simulink model "CubeSat_Archiv"  (R2019a)
settings: Solver=VariableStepAuto  StartTime=0.0  StopTime=10.0  RelTol=1e-3
undefined symbols (not defined in the file): D_distri, G_g, G_s, G_t, Gs, I_rw, I_vscmg, I_w, J_w, Kc, Ki, Kp, Kv, Kw_d, Kw_i, Kw_p, m, OMEGA_0, quat_0, smiData, tau_sat_mt, w_rw_ref, X, Y, Z
libraries: sm_lib x57, nesl_utility x28, aerolibutil x18, sharedtransform x5, ADCS_lib x4, simulink x2, sharedutil x2
(part 4 of 4)

== system CubeSat_Archiv/Simscape Plant/Simscape Plant1/CubeSat Structure ==
  BODY_FIXED_CoMXform : sm_lib/Frames and Transforms/Rigid Transform  TranslationMethod=Cartesian  TranslationStandardOffset=0  TranslationLengthUnit=mm  TranslationStandardAxis=+Z  TranslationCartesianOffset=smiData.RigidTransform(10).translation  TranslationROffset=0  TranslationROffsetUnits=m  TranslationZOffset=0  TranslationZOffsetUnits=m  TranslationThetaOffset=0  TranslationThetaOffsetUnits=deg  RotationMethod=ArbitraryAxis  RotationAngleUnits=rad  RotationStandardAxis=+Z  RotationAngle=smiData.RigidTransform(10).angle  RotationArbitraryAxis=smiData.RigidTransform(10).axis  FollAlignAxisA=+X  BaseAlignAxisA=+Y  FollAlignAxisB=+Y  BaseAlignAxisB=+Z  RotationSequenceAxes=FollowerAxes  RotationSequence=XYX  RotationSequenceAngles=[0 0 0]  RotationSequenceAnglesUnits=deg  RotationMatrix=[1 0 0; 0 1 0; 0 0 1]
  ReferenceFrame : sm_lib/Frames and Transforms/Reference Frame
  Solid : sm_lib/Body Elements/Solid  InertiaType=Custom  Mass=smiData.Solid(1).mass  MassUnits=kg  CenterOfMass=smiData.Solid(1).CoM  CenterOfMassUnits=mm  MomentsOfInertia=smiData.Solid(1).MoI  MomentsOfInertiaUnits=kg*mm^2  ProductsOfInertia=smiData.Solid(1).PoI  ProductsOfInertiaUnits=kg*mm^2  BasedOnType=Density  Density=1000  DensityUnits=kg/m^3  DoExposeReferenceFrame=on  SerializedFrames=<Frames><Frame><Id>Frame1</Id><Value><Name>F1</Name><Origin><Source>CenterOfMassFrame</Source><FeatureName></FeatureName></Origin><PrimaryAxis><DefinedDirection>+Z</DefinedDirection><Source>ReferenceFrame</Source><SourceDirection>+Z</SourceDirection><FeatureName></FeatureName></PrimaryAxis><SecondaryAxis><DefinedDirection>+X</DefinedDirection><Source>ReferenceFrame</Source><SourceDirection>+X</SourceDirection><FeatureName></FeatureName></SecondaryAxis></Value></Frame></Frames>  GraphicType=FromGeometry  MarkerShape=Sphere  MarkerSize=10  GraphicVisPropType=SimpleVisualProperties  GraphicDiffuseColor=[0.6 0.6 0.6]  GraphicSpecularColor=[0.5 0.5 0.5 1.0]  GraphicAmbientColor=[0.15 0.15 0.15 1.0]  GraphicEmissiveColor=[0.0 0.0 0.0 1.0]  GraphicShininess=100  GraphicOpacity=smiData.Solid(1).opacity  GeometryShape=FromFile  RectangleSize=[1 1]  RectangleSizeUnits=m  BrickDimensions=[1 1 1]  BrickDimensionUnits=m  CylinderRadius=1  CylinderRadiusUnits=m  CylinderLength=1  CylinderLengthUnits=m  SphereRadius=1  SphereRadiusUnits=m  EllipsoidRadii=[1 1 1]  EllipsoidRadiiUnits=m  ExtrusionCrossSection=[1 1; -1 1; -1 -1; 1 -1]  ExtrusionCrossSectionUnits=m  ExtrusionLength=1  ExtrusionLengthUnits=m  PolygonNumSides=3  PolygonOuterRadius=1  PolygonOuterRadiusUnits=m  ExtGeomFileType=STEP  ExtGeomFileName=body_part_acis_Default_sldprt.STEP  ExtGeomFileUnits=m  RevolutionCrossSection=[1 1; 1 -1; 2 -1; 2 1]  RevolutionCrossSectionUnits=m  RevolutionExtent=Full  RevolutionAngle=180  RevolutionAngleUnits=deg
  Transform : sm_lib/Frames and Transforms/Rigid Transform  TranslationMethod=Cartesian  TranslationStandardOffset=0  TranslationLengthUnit=mm  TranslationStandardAxis=+Z  TranslationCartesianOffset=smiData.RigidTransform(1).translation  TranslationROffset=0  TranslationROffsetUnits=m  TranslationZOffset=0  TranslationZOffsetUnits=m  TranslationThetaOffset=0  TranslationThetaOffsetUnits=deg  RotationMethod=ArbitraryAxis  RotationAngleUnits=rad  RotationStandardAxis=+Z  RotationAngle=smiData.RigidTransform(1).angle  RotationArbitraryAxis=smiData.RigidTransform(1).axis  FollAlignAxisA=+X  BaseAlignAxisA=+Y  FollAlignAxisB=+Y  BaseAlignAxisB=+Z  RotationSequenceAxes=FollowerAxes  RotationSequence=XYX  RotationSequenceAngles=[0 0 0]  RotationSequenceAnglesUnits=deg  RotationMatrix=[1 0 0; 0 1 0; 0 0 1]
  Transform1 : sm_lib/Frames and Transforms/Rigid Transform  TranslationMethod=Cartesian  TranslationStandardOffset=0  TranslationLengthUnit=mm  TranslationStandardAxis=+Z  TranslationCartesianOffset=smiData.RigidTransform(3).translation  TranslationROffset=0  TranslationROffsetUnits=m  TranslationZOffset=0  TranslationZOffsetUnits=m  TranslationThetaOffset=0  TranslationThetaOffsetUnits=deg  RotationMethod=ArbitraryAxis  RotationAngleUnits=rad  RotationStandardAxis=+Z  RotationAngle=smiData.RigidTransform(3).angle  RotationArbitraryAxis=smiData.RigidTransform(3).axis  FollAlignAxisA=+X  BaseAlignAxisA=+Y  FollAlignAxisB=+Y  BaseAlignAxisB=+Z  RotationSequenceAxes=FollowerAxes  RotationSequence=XYX  RotationSequenceAngles=[0 0 0]  RotationSequenceAnglesUnits=deg  RotationMatrix=[1 0 0; 0 1 0; 0 0 1]
  Transform2 : sm_lib/Frames and Transforms/Rigid Transform  TranslationMethod=Cartesian  TranslationStandardOffset=0  TranslationLengthUnit=mm  TranslationStandardAxis=+Z  TranslationCartesianOffset=smiData.RigidTransform(5).translation  TranslationROffset=0  TranslationROffsetUnits=m  TranslationZOffset=0  TranslationZOffsetUnits=m  TranslationThetaOffset=0  TranslationThetaOffsetUnits=deg  RotationMethod=ArbitraryAxis  RotationAngleUnits=rad  RotationStandardAxis=+Z  RotationAngle=smiData.RigidTransform(5).angle  RotationArbitraryAxis=smiData.RigidTransform(5).axis  FollAlignAxisA=+X  BaseAlignAxisA=+Y  FollAlignAxisB=+Y  BaseAlignAxisB=+Z  RotationSequenceAxes=FollowerAxes  RotationSequence=XYX  RotationSequenceAngles=[0 0 0]  RotationSequenceAnglesUnits=deg  RotationMatrix=[1 0 0; 0 1 0; 0 0 1]
  Transform3 : sm_lib/Frames and Transforms/Rigid Transform  TranslationMethod=Cartesian  TranslationStandardOffset=0  TranslationLengthUnit=mm  TranslationStandardAxis=+Z  TranslationCartesianOffset=smiData.RigidTransform(7).translation  TranslationROffset=0  TranslationROffsetUnits=m  TranslationZOffset=0  TranslationZOffsetUnits=m  TranslationThetaOffset=0  TranslationThetaOffsetUnits=deg  RotationMethod=ArbitraryAxis  RotationAngleUnits=rad  RotationStandardAxis=+Z  RotationAngle=smiData.RigidTransform(7).angle  RotationArbitraryAxis=smiData.RigidTransform(7).axis  FollAlignAxisA=+X  BaseAlignAxisA=+Y  FollAlignAxisB=+Y  BaseAlignAxisB=+Z  RotationSequenceAxes=FollowerAxes  RotationSequence=XYX  RotationSequenceAngles=[0 0 0]  RotationSequenceAnglesUnits=deg  RotationMatrix=[1 0 0; 0 1 0; 0 0 1]
  CoM : PMIOPort  Side=Left
  F3 : PMIOPort  Port=2  Side=Right
  F2 : PMIOPort  Port=3  Side=Right
  F1 : PMIOPort  Port=4  Side=Right
  F : PMIOPort  Port=5  Side=Right
  connections:
  BODY_FIXED_CoMXform/LConn1 -- CoM/RConn1
  Transform3/RConn1 -- F3/RConn1
  Transform2/RConn1 -- F2/RConn1
  Transform1/RConn1 -- F1/RConn1
  Transform/RConn1 -- F/RConn1
  Transform2/LConn1 -- BODY_FIXED_CoMXform/RConn1 -- Transform3/LConn1 -- ReferenceFrame/RConn1 -- Solid/RConn1 -- Transform1/LConn1 -- Transform/LConn1

== system CubeSat_Archiv/Simscape Plant/Simscape Plant1/RW 1 Disk ==
  ReferenceFrame : sm_lib/Frames and Transforms/Reference Frame
  Solid : sm_lib/Body Elements/Solid  InertiaType=Custom  Mass=smiData.Solid(2).mass  MassUnits=kg  CenterOfMass=smiData.Solid(2).CoM  CenterOfMassUnits=mm  MomentsOfInertia=smiData.Solid(2).MoI  MomentsOfInertiaUnits=kg*mm^2  ProductsOfInertia=smiData.Solid(2).PoI  ProductsOfInertiaUnits=kg*mm^2  BasedOnType=Density  Density=1000  DensityUnits=kg/m^3  DoExposeReferenceFrame=on  SerializedFrames=<Frames/>  GraphicType=FromGeometry  MarkerShape=Sphere  MarkerSize=10  GraphicVisPropType=SimpleVisualProperties  GraphicDiffuseColor=smiData.Solid(2).color  GraphicSpecularColor=[0.5 0.5 0.5 1.0]  GraphicAmbientColor=[0.15 0.15 0.15 1.0]  GraphicEmissiveColor=[0.0 0.0 0.0 1.0]  GraphicShininess=75  GraphicOpacity=smiData.Solid(2).opacity  GeometryShape=FromFile  RectangleSize=[1 1]  RectangleSizeUnits=m  BrickDimensions=[1 1 1]  BrickDimensionUnits=m  CylinderRadius=1  CylinderRadiusUnits=m  CylinderLength=1  CylinderLengthUnits=m  SphereRadius=1  SphereRadiusUnits=m  EllipsoidRadii=[1 1 1]  EllipsoidRadiiUnits=m  ExtrusionCrossSection=[1 1; -1 1; -1 -1; 1 -1]  ExtrusionCrossSectionUnits=m  ExtrusionLength=1  ExtrusionLengthUnits=m  PolygonNumSides=3  PolygonOuterRadius=1  PolygonOuterRadiusUnits=m  ExtGeomFileType=STEP  ExtGeomFileName=wheel_part_acis_Default_sldprt.STEP  ExtGeomFileUnits=m  RevolutionCrossSection=[1 1; 1 -1; 2 -1; 2 1]  RevolutionCrossSectionUnits=m  RevolutionExtent=Full  RevolutionAngle=180  RevolutionAngleUnits=deg
  Transform : sm_lib/Frames and Transforms/Rigid Transform  TranslationMethod=Cartesian  TranslationStandardOffset=0  TranslationLengthUnit=mm  TranslationStandardAxis=+Z  TranslationCartesianOffset=smiData.RigidTransform(4).translation  TranslationROffset=0  TranslationROffsetUnits=m  TranslationZOffset=0  TranslationZOffsetUnits=m  TranslationThetaOffset=0  TranslationThetaOffsetUnits=deg  RotationMethod=ArbitraryAxis  RotationAngleUnits=rad  RotationStandardAxis=+Z  RotationAngle=smiData.RigidTransform(4).angle  RotationArbitraryAxis=smiData.RigidTransform(4).axis  FollAlignAxisA=+X  BaseAlignAxisA=+Y  FollAlignAxisB=+Y  BaseAlignAxisB=+Z  RotationSequenceAxes=FollowerAxes  RotationSequence=XYX  RotationSequenceAngles=[0 0 0]  RotationSequenceAnglesUnits=deg  RotationMatrix=[1 0 0; 0 1 0; 0 0 1]
  F : PMIOPort  Side=Left
  connections:
  Transform/RConn1 -- F/RConn1
  Transform/LConn1 -- Solid/RConn1 -- ReferenceFrame/RConn1

== system CubeSat_Archiv/Simscape Plant/Simscape Plant1/RW 2 Disk ==
  ReferenceFrame : sm_lib/Frames and Transforms/Reference Frame
  Solid : sm_lib/Body Elements/Solid  InertiaType=Custom  Mass=smiData.Solid(2).mass  MassUnits=kg  CenterOfMass=smiData.Solid(2).CoM  CenterOfMassUnits=mm  MomentsOfInertia=smiData.Solid(2).MoI  MomentsOfInertiaUnits=kg*mm^2  ProductsOfInertia=smiData.Solid(2).PoI  ProductsOfInertiaUnits=kg*mm^2  BasedOnType=Density  Density=1000  DensityUnits=kg/m^3  DoExposeReferenceFrame=on  SerializedFrames=<Frames/>  GraphicType=FromGeometry  MarkerShape=Sphere  MarkerSize=10  GraphicVisPropType=SimpleVisualProperties  GraphicDiffuseColor=smiData.Solid(2).color  GraphicSpecularColor=[0.5 0.5 0.5 1.0]  GraphicAmbientColor=[0.15 0.15 0.15 1.0]  GraphicEmissiveColor=[0.0 0.0 0.0 1.0]  GraphicShininess=75  GraphicOpacity=smiData.Solid(2).opacity  GeometryShape=FromFile  RectangleSize=[1 1]  RectangleSizeUnits=m  BrickDimensions=[1 1 1]  BrickDimensionUnits=m  CylinderRadius=1  CylinderRadiusUnits=m  CylinderLength=1  CylinderLengthUnits=m  SphereRadius=1  SphereRadiusUnits=m  EllipsoidRadii=[1 1 1]  EllipsoidRadiiUnits=m  ExtrusionCrossSection=[1 1; -1 1; -1 -1; 1 -1]  ExtrusionCrossSectionUnits=m  ExtrusionLength=1  ExtrusionLengthUnits=m  PolygonNumSides=3  PolygonOuterRadius=1  PolygonOuterRadiusUnits=m  ExtGeomFileType=STEP  ExtGeomFileName=wheel_part_acis_Default_sldprt.STEP  ExtGeomFileUnits=m  RevolutionCrossSection=[1 1; 1 -1; 2 -1; 2 1]  RevolutionCrossSectionUnits=m  RevolutionExtent=Full  RevolutionAngle=180  RevolutionAngleUnits=deg
  Transform : sm_lib/Frames and Transforms/Rigid Transform  TranslationMethod=Cartesian  TranslationStandardOffset=0  TranslationLengthUnit=mm  TranslationStandardAxis=+Z  TranslationCartesianOffset=smiData.RigidTransform(6).translation  TranslationROffset=0  TranslationROffsetUnits=m  TranslationZOffset=0  TranslationZOffsetUnits=m  TranslationThetaOffset=0  TranslationThetaOffsetUnits=deg  RotationMethod=ArbitraryAxis  RotationAngleUnits=rad  RotationStandardAxis=+Z  RotationAngle=smiData.RigidTransform(6).angle  RotationArbitraryAxis=smiData.RigidTransform(6).axis  FollAlignAxisA=+X  BaseAlignAxisA=+Y  FollAlignAxisB=+Y  BaseAlignAxisB=+Z  RotationSequenceAxes=FollowerAxes  RotationSequence=XYX  RotationSequenceAngles=[0 0 0]  RotationSequenceAnglesUnits=deg  RotationMatrix=[1 0 0; 0 1 0; 0 0 1]
  F : PMIOPort  Side=Left
  connections:
  Transform/RConn1 -- F/RConn1
  Transform/LConn1 -- Solid/RConn1 -- ReferenceFrame/RConn1

== system CubeSat_Archiv/Simscape Plant/Simscape Plant1/RW 3 Disk ==
  ReferenceFrame : sm_lib/Frames and Transforms/Reference Frame
  Solid : sm_lib/Body Elements/Solid  InertiaType=Custom  Mass=smiData.Solid(2).mass  MassUnits=kg  CenterOfMass=smiData.Solid(2).CoM  CenterOfMassUnits=mm  MomentsOfInertia=smiData.Solid(2).MoI  MomentsOfInertiaUnits=kg*mm^2  ProductsOfInertia=smiData.Solid(2).PoI  ProductsOfInertiaUnits=kg*mm^2  BasedOnType=Density  Density=1000  DensityUnits=kg/m^3  DoExposeReferenceFrame=on  SerializedFrames=<Frames/>  GraphicType=FromGeometry  MarkerShape=Sphere  MarkerSize=10  GraphicVisPropType=SimpleVisualProperties  GraphicDiffuseColor=smiData.Solid(2).color  GraphicSpecularColor=[0.5 0.5 0.5 1.0]  GraphicAmbientColor=[0.15 0.15 0.15 1.0]  GraphicEmissiveColor=[0.0 0.0 0.0 1.0]  GraphicShininess=75  GraphicOpacity=smiData.Solid(2).opacity  GeometryShape=FromFile  RectangleSize=[1 1]  RectangleSizeUnits=m  BrickDimensions=[1 1 1]  BrickDimensionUnits=m  CylinderRadius=1  CylinderRadiusUnits=m  CylinderLength=1  CylinderLengthUnits=m  SphereRadius=1  SphereRadiusUnits=m  EllipsoidRadii=[1 1 1]  EllipsoidRadiiUnits=m  ExtrusionCrossSection=[1 1; -1 1; -1 -1; 1 -1]  ExtrusionCrossSectionUnits=m  ExtrusionLength=1  ExtrusionLengthUnits=m  PolygonNumSides=3  PolygonOuterRadius=1  PolygonOuterRadiusUnits=m  ExtGeomFileType=STEP  ExtGeomFileName=wheel_part_acis_Default_sldprt.STEP  ExtGeomFileUnits=m  RevolutionCrossSection=[1 1; 1 -1; 2 -1; 2 1]  RevolutionCrossSectionUnits=m  RevolutionExtent=Full  RevolutionAngle=180  RevolutionAngleUnits=deg
  Transform : sm_lib/Frames and Transforms/Rigid Transform  TranslationMethod=Cartesian  TranslationStandardOffset=0  TranslationLengthUnit=mm  TranslationStandardAxis=+Z  TranslationCartesianOffset=smiData.RigidTransform(8).translation  TranslationROffset=0  TranslationROffsetUnits=m  TranslationZOffset=0  TranslationZOffsetUnits=m  TranslationThetaOffset=0  TranslationThetaOffsetUnits=deg  RotationMethod=ArbitraryAxis  RotationAngleUnits=rad  RotationStandardAxis=+Z  RotationAngle=smiData.RigidTransform(8).angle  RotationArbitraryAxis=smiData.RigidTransform(8).axis  FollAlignAxisA=+X  BaseAlignAxisA=+Y  FollAlignAxisB=+Y  BaseAlignAxisB=+Z  RotationSequenceAxes=FollowerAxes  RotationSequence=XYX  RotationSequenceAngles=[0 0 0]  RotationSequenceAnglesUnits=deg  RotationMatrix=[1 0 0; 0 1 0; 0 0 1]
  F : PMIOPort  Side=Left
  connections:
  Transform/RConn1 -- F/RConn1
  Transform/LConn1 -- Solid/RConn1 -- ReferenceFrame/RConn1

== system CubeSat_Archiv/Simscape Plant/Simscape Plant1/RW 4 Disk ==
  ReferenceFrame : sm_lib/Frames and Transforms/Reference Frame
  Solid : sm_lib/Body Elements/Solid  InertiaType=Custom  Mass=smiData.Solid(2).mass  MassUnits=kg  CenterOfMass=smiData.Solid(2).CoM  CenterOfMassUnits=mm  MomentsOfInertia=smiData.Solid(2).MoI  MomentsOfInertiaUnits=kg*mm^2  ProductsOfInertia=smiData.Solid(2).PoI  ProductsOfInertiaUnits=kg*mm^2  BasedOnType=Density  Density=1000  DensityUnits=kg/m^3  DoExposeReferenceFrame=on  SerializedFrames=<Frames/>  GraphicType=FromGeometry  MarkerShape=Sphere  MarkerSize=10  GraphicVisPropType=SimpleVisualProperties  GraphicDiffuseColor=smiData.Solid(2).color  GraphicSpecularColor=[0.5 0.5 0.5 1.0]  GraphicAmbientColor=[0.15 0.15 0.15 1.0]  GraphicEmissiveColor=[0.0 0.0 0.0 1.0]  GraphicShininess=75  GraphicOpacity=smiData.Solid(2).opacity  GeometryShape=FromFile  RectangleSize=[1 1]  RectangleSizeUnits=m  BrickDimensions=[1 1 1]  BrickDimensionUnits=m  CylinderRadius=1  CylinderRadiusUnits=m  CylinderLength=1  CylinderLengthUnits=m  SphereRadius=1  SphereRadiusUnits=m  EllipsoidRadii=[1 1 1]  EllipsoidRadiiUnits=m  ExtrusionCrossSection=[1 1; -1 1; -1 -1; 1 -1]  ExtrusionCrossSectionUnits=m  ExtrusionLength=1  ExtrusionLengthUnits=m  PolygonNumSides=3  PolygonOuterRadius=1  PolygonOuterRadiusUnits=m  ExtGeomFileType=STEP  ExtGeomFileName=wheel_part_acis_Default_sldprt.STEP  ExtGeomFileUnits=m  RevolutionCrossSection=[1 1; 1 -1; 2 -1; 2 1]  RevolutionCrossSectionUnits=m  RevolutionExtent=Full  RevolutionAngle=180  RevolutionAngleUnits=deg
  Transform : sm_lib/Frames and Transforms/Rigid Transform  TranslationMethod=Cartesian  TranslationStandardOffset=0  TranslationLengthUnit=mm  TranslationStandardAxis=+Z  TranslationCartesianOffset=smiData.RigidTransform(2).translation  TranslationROffset=0  TranslationROffsetUnits=m  TranslationZOffset=0  TranslationZOffsetUnits=m  TranslationThetaOffset=0  TranslationThetaOffsetUnits=deg  RotationMethod=ArbitraryAxis  RotationAngleUnits=rad  RotationStandardAxis=+Z  RotationAngle=smiData.RigidTransform(2).angle  RotationArbitraryAxis=smiData.RigidTransform(2).axis  FollAlignAxisA=+X  BaseAlignAxisA=+Y  FollAlignAxisB=+Y  BaseAlignAxisB=+Z  RotationSequenceAxes=FollowerAxes  RotationSequence=XYX  RotationSequenceAngles=[0 0 0]  RotationSequenceAnglesUnits=deg  RotationMatrix=[1 0 0; 0 1 0; 0 0 1]
  F : PMIOPort  Side=Left
  connections:
  Transform/RConn1 -- F/RConn1
  Transform/LConn1 -- Solid/RConn1 -- ReferenceFrame/RConn1

== system CubeSat_Archiv/vscmg dynamics v1.0/Dynamics VSCMG/omega_g ==
  OMEGA : Inport
  Gain : Gain  Gain=transpose(G_g(:,1))  Multiplication=Matrix(K*u)
  Gain1 : Gain  Gain=transpose(G_g(:,2))  Multiplication=Matrix(K*u)
  Gain2 : Gain  Gain=transpose(G_g(:,3))  Multiplication=Matrix(K*u)
  Gain3 : Gain  Gain=transpose(G_g(:,4))  Multiplication=Matrix(K*u)
  Mux : Mux
  omega_g : Outport
  wires:
  Mux/1 -> omega_g/1
  Gain3/1 -> Mux/4
  Gain2/1 -> Mux/3
  Gain1/1 -> Mux/2
  Gain/1 -> Mux/1
  OMEGA/1 -> Gain/1, Gain1/1, Gain2/1, Gain3/1

== system CubeSat_Archiv/vscmg dynamics v1.0/Dynamics VSCMG/omega_t ==
  OMEGA : Inport
  Gain : Gain  Gain=transpose(G_t(:,1))  Multiplication=Matrix(K*u)
  Gain1 : Gain  Gain=transpose(G_t(:,2))  Multiplication=Matrix(K*u)
  Gain2 : Gain  Gain=transpose(G_t(:,3))  Multiplication=Matrix(K*u)
  Gain3 : Gain  Gain=transpose(G_t(:,4))  Multiplication=Matrix(K*u)
  Mux : Mux
  omega_t : Outport
  wires:
  OMEGA/1 -> Gain3/1, Gain2/1, Gain1/1, Gain/1
  Gain/1 -> Mux/1
  Gain1/1 -> Mux/2
  Gain2/1 -> Mux/3
  Gain3/1 -> Mux/4
  Mux/1 -> omega_t/1

== system CubeSat_Archiv/vscmg dynamics v1.0/VSCMGC/RW 1 ==
  ALPHA : Inport
  u_s_1 : Inport  Port=2
  Gain : Gain  Gain=1/I_w(1,1)
  Gain1 : Gain  Gain=G_s(:,1).'  Multiplication=Matrix(K*u)
  Integrator : Integrator
  Sum : Sum  Inputs=+-
  omega_w_1 : Outport
  alpha_w_1 : Outport  Port=2
  wires:
  Sum/1 -> alpha_w_1/1, Integrator/1
  Integrator/1 -> omega_w_1/1
  u_s_1/1 -> Gain/1
  Gain/1 -> Sum/1
  Gain1/1 -> Sum/2
  ALPHA/1 -> Gain1/1

== system CubeSat_Archiv/vscmg dynamics v1.0/VSCMGC/RW 2 ==
  ALPHA : Inport
  u_s_2 : Inport  Port=2
  Gain : Gain  Gain=1/I_w(1,2)
  Gain1 : Gain  Gain=G_s(:,2).'  Multiplication=Matrix(K*u)
  Integrator : Integrator
  Sum : Sum  Inputs=+-
  omega_w_2 : Outport
  alpha_w_2 : Outport  Port=2
  wires:
  ALPHA/1 -> Gain1/1
  Gain1/1 -> Sum/2
  Gain/1 -> Sum/1
  u_s_2/1 -> Gain/1
  Integrator/1 -> omega_w_2/1
  Sum/1 -> alpha_w_2/1, Integrator/1

== system CubeSat_Archiv/vscmg dynamics v1.0/VSCMGC/RW 3 ==
  ALPHA : Inport
  u_s_3 : Inport  Port=2
  Gain : Gain  Gain=1/I_w(1,3)
  Gain1 : Gain  Gain=G_s(:,3).'  Multiplication=Matrix(K*u)
  Integrator : Integrator
  Sum : Sum  Inputs=+-
  omega_w_3 : Outport
  alpha_w_3 : Outport  Port=2
  wires:
  Sum/1 -> alpha_w_3/1, Integrator/1
  Integrator/1 -> omega_w_3/1
  u_s_3/1 -> Gain/1
  Gain/1 -> Sum/1
  Gain1/1 -> Sum/2
  ALPHA/1 -> Gain1/1

== system CubeSat_Archiv/vscmg dynamics v1.0/VSCMGC/RW 4 ==
  ALPHA : Inport
  u_s_4 : Inport  Port=2
  Gain : Gain  Gain=1/I_w(1,4)
  Gain1 : Gain  Gain=G_s(:,4).'  Multiplication=Matrix(K*u)
  Integrator : Integrator
  Sum : Sum  Inputs=+-
  omega_w_4 : Outport
  alpha_w_4 : Outport  Port=2
  wires:
  ALPHA/1 -> Gain1/1
  Gain1/1 -> Sum/2
  Gain/1 -> Sum/1
  u_s_4/1 -> Gain/1
  Integrator/1 -> omega_w_4/1
  Sum/1 -> alpha_w_4/1, Integrator/1

== system CubeSat_Archiv/Controller1/LQI_Full State_Verified1/Vector Out Unwinding1/Short Rotation ==
  q : Inport
  Gain1 : Gain  Gain=-1
  Sign1 : Signum
  extract scalar part : Selector  InputPortWidth=4  IndexOptions=Index vector (dialog)  Indices=[1]  OutputSizes=1
  sgn : Outport
  wires:
  q/1 -> extract scalar part/1
  extract scalar part/1 -> Sign1/1
  Sign1/1 -> Gain1/1
  Gain1/1 -> sgn/1

== matlab function CubeSat_Archiv/Simscape Plant/FeedFwd/Vector Cross Product ==
  data: u input; u_tilde output
function u_tilde = tilde(u)
u_tilde = [0 -u(3) u(2);
           u(3) 0 -u(1);
           -u(2) u(1) 0];

== matlab function CubeSat_Archiv/Simscape Plant/FeedFwd/Vector Cross Product1 ==
  data: u input; u_tilde output
function u_tilde = tilde(u)
u_tilde = [0 -u(3,1) u(2,1);
           u(3,1) 0 -u(1,1);
           -u(2,1) u(1,1) 0];

== matlab function CubeSat_Archiv/QuEST ==
  data: V_N input; BN output size=[4 1]; V_B input; WT input
function BN = quest(V_N,V_B,WT)
B = zeros(3);

% count # of sensors
dim = size(V_N); 
n_sensor = dim(2);

% normalize V_N
for n = 1:n_sensor
    V_N(:,n)=V_N(:,n)/norm(V_N(:,n));
end
    
% normalize V_B
for n = 1:n_sensor
    V_B(:,n)=V_B(:,n)/norm(V_B(:,n));
end

% assemble K matrix
for n = 1:n_sensor
    B=WT(n)*V_B(:,n)*transpose(V_N(:,n))+B;
end
S = B+transpose(B);
sigma = trace(B);
Z = [B(2,3)-B(3,2);
     B(3,1)-B(1,3);
     B(1,2)-B(2,1)];
K = [sigma transpose(Z);Z S-sigma*eye(3)];

% optimize eigenvalue
lambda = sum(WT); % first guess
for i = 1:2
    f = det(K-lambda*eye(4));
    f_dash = det(K-lambda*eye(4))*trace(inv(K-lambda*eye(4))*-eye(4));
    lambda = lambda - (f/f_dash);
end

% compute Rodrigues parameter & convert to Quaternion
q = inv((lambda+sigma)*eye(3)-S)*Z;
quatr = [1;q]/sqrt(1+transpose(q)*q);

BN = quatr;

== matlab function CubeSat_Archiv/Reaction Wheel ==
  data: ALPHA input; tau_wheel output; u_s_cmd input; index input; omega_wheel output; h_wheel output
function [tau_wheel,omega_wheel,h_wheel] = RW(ALPHA,u_s_cmd,index)

tau_wheel = u_s_cmd-J_w(1,index)*(transpose(Gs(:,index))*ALPHA);
omega_wheel = (tau_wheel^2)/(2*J_w(1,index));
h_wheel = J_w(1,index)*omega_wheel;

== matlab function CubeSat_Archiv/Reaction Wheel Cluster/Reaction Wheel 1 ==
  data: ALPHA input; tau_wheel output; u_s_cmd input; index input; omega_wheel output; h_wheel output
function [tau_wheel,omega_wheel,h_wheel] = RW(ALPHA,u_s_cmd,index)

tau_wheel = u_s_cmd-J_w(1,index)*(transpose(Gs(:,index))*ALPHA);
omega_wheel = (tau_wheel^2)/(2*J_w(1,index));
h_wheel = J_w(1,index)*omega_wheel;

== matlab function CubeSat_Archiv/Reaction Wheel Cluster/Reaction Wheel 2 ==
  data: ALPHA input; tau_wheel output; u_s_cmd input; index input; omega_wheel output; h_wheel output
function [tau_wheel,omega_wheel,h_wheel] = RW(ALPHA,u_s_cmd,index)

tau_wheel = u_s_cmd-J_w(1,index)*(transpose(Gs(:,index))*ALPHA);
omega_wheel = (tau_wheel^2)/(2*J_w(1,index));
h_wheel = J_w(1,index)*omega_wheel;

== matlab function CubeSat_Archiv/Reaction Wheel Cluster/Reaction Wheel 3 ==
  data: ALPHA input; tau_wheel output; u_s_cmd input; index input; omega_wheel output; h_wheel output
function [tau_wheel,omega_wheel,h_wheel] = RW(ALPHA,u_s_cmd,index)

tau_wheel = u_s_cmd-J_w(1,index)*(transpose(Gs(:,index))*ALPHA);
omega_wheel = (tau_wheel^2)/(2*J_w(1,index));
h_wheel = J_w(1,index)*omega_wheel;

== matlab function CubeSat_Archiv/Reaction Wheel Cluster/Reaction Wheel 4 ==
  data: ALPHA input; tau_wheel output; u_s_cmd input; index input; omega_wheel output; h_wheel output
function [tau_wheel,omega_wheel,h_wheel] = RW(ALPHA,u_s_cmd,index)

tau_wheel = u_s_cmd-J_w(1,index)*(transpose(Gs(:,index))*ALPHA);
omega_wheel = (tau_wheel^2)/(2*J_w(1,index));
h_wheel = J_w(1,index)*omega_wheel;

== matlab function CubeSat_Archiv/Satellite Dynamics/Equation of Motion ==
  data: OMEGA input; ALPHA output; h_app_RWC input; tau_app_RWC input; tau_app_distrb input
function ALPHA = dynamics(OMEGA,h_app_RWC,tau_app_RWC,tau_app_distrb)

% assemble OMEGA_tilde for cross product
OMEGA_tilde = [0 -OMEGA(3) OMEGA(2);
               OMEGA(3) 0 -OMEGA(1);
              -OMEGA(2) OMEGA(1) 0];
          
% calculate ALPHA
ALPHA = inv(I_tot) * (-OMEGA_tilde*I_tot*OMEGA - tau_app_RWC - OMEGA_tilde*h_app_RWC + tau_app_distrb)

== matlab function CubeSat_Archiv/Dynamics/Vector Cross Product ==
  data: u input; u_tilde output
function u_tilde = tilde(u)
u_tilde = [0 -u(3) u(2);
           u(3) 0 -u(1);
           -u(2) u(1) 0];

== matlab function CubeSat_Archiv/Dynamics/Vector Cross Product1 ==
  data: u input; u_tilde output
function u_tilde = tilde(u)
u_tilde = [0 -u(3,1) u(2,1);
           u(3,1) 0 -u(1,1);
           -u(2,1) u(1,1) 0];

== matlab function CubeSat_Archiv/tilde_cross P ==
  data: u input; u_tilde output
function u_tilde = tilde(u)
u_tilde = [0 -u(3) u(2);
           u(3) 0 -u(1);
           -u(2) u(1) 0];

== matlab function CubeSat_Archiv/FeedFwd/Vector Cross Product ==
  data: u input; u_tilde output
function u_tilde = tilde(u)
u_tilde = [0 -u(3) u(2);
           u(3) 0 -u(1);
           -u(2) u(1) 0];

== matlab function CubeSat_Archiv/vscmg dynamics v1.0/Dynamics VSCMG/Vector Cross Product ==
  data: u input; u_tilde output
function u_tilde = tilde(u)
u_tilde = [0 -u(3) u(2);
           u(3) 0 -u(1);
           -u(2) u(1) 0];

== matlab function CubeSat_Archiv/FeedFwd/Vector Cross Product1 ==
  data: u input; u_tilde output
function u_tilde = tilde(u)
u_tilde = [0 -u(3,1) u(2,1);
           u(3,1) 0 -u(1,1);
           -u(2,1) u(1,1) 0];

== matlab function CubeSat_Archiv/Dynamics without FF/Vector Cross Product ==
  data: u input; u_tilde output
function u_tilde = tilde(u)
u_tilde = [0 -u(3) u(2);
           u(3) 0 -u(1);
           -u(2) u(1) 0];

== matlab function CubeSat_Archiv/PIV Full EoM_Verified/Cross Product ==
  data: u input; u_tilde output
function u_tilde = tilde(u)
u_tilde = [0 -u(3) u(2);
           u(3) 0 -u(1);
           -u(2) u(1) 0];

== matlab function CubeSat_Archiv/Dynamics without FF/Vector Cross Product1 ==
  data: u input; u_tilde output
function u_tilde = tilde(u)
u_tilde = [0 -u(3,1) u(2,1);
           u(3,1) 0 -u(1,1);
           -u(2,1) u(1,1) 0];
